simulink model "GridFormingConverter"  (R2024b)
settings: Solver=ode1be  StartTime=0.0  StopTime=simulationTime  FixedStep=gridInverter.vsm.samplingTime  MaxStep=gridInverter.vsm.samplingTime  RelTol=1e-3  AbsTol=1e-3
PreLoadFcn:
  | % Parameterize the model
  | GridFormingConverterInputParameters;
PostLoadFcn:
  | GridFormingConverterTestCondition;
undefined symbols (not defined in the file): base, DiscIntNeverNeededParam, grid, gridInverter, localSolverSampleTime, scrFactorRg, scrFactorXg, transformer, TransmissionLine
libraries: ee_lib x15, eeGeneralControl x15, nesl_utility x11, simulink x5, fl_lib x4, eeTransforms x4, batteryecm_lib x1, eeSinGeneratorThreePhase x1, simulink_extras x1, eePowerMeasurement x1
(part 1 of 3)
CloseFcn:
  | try, close( 'GridFormingConverterNormalOperation'), end
  | try, close( 'GridFormingConverterActivePowerChange'), end
  | try, close( 'GridFormingConverterReactivePowerChange'), end
  | try, close( 'GridFormingConverterGridVoltageChange'), end
  | try, close( 'GridFormingConverterLocalLoadChange'), end
  | try, close( 'GridFormingConverterSmallGridFreqChange'), end
  | try, close( 'GridFormingConverterLargeGridFreqChange'), end
  | try, close( 'GridFormingConverterFullGridFreqChange'), end
  | try, close( 'GridFormingConverter10DegGridPhaseChange'), end
  | try, close( 'GridFormingConverter60DegGridPhaseChange'), end
  | try, close( 'GridFormingConverterPermanentFault'), end
  | try, close( 'GridFormingConverterTemporaryFault'), end
  | try, close( 'GridFormingConverterActivePowerChangeWithRipple'), end
  | try, close( 'GridFormingConverterIslanding'), end
  | try, close( 'GridFormingConverterDampingEffect'), end
  | try, close( 'GridFormingConverterIntertiaEffect'), end
  | try, close('GridFormingConverterVdControllerBodePlot'), end
  | try, close('GridFormingConverterControllerBodePlot'), end
  | try, close( 'GridFormingConverterThreePhaseFault'), end
  | try, close( 'GridFormingConverterThreePhaseFaultStandard'), end
  | try, close( 'GridFormingConverterCompareFaultRideMethod'), end
  | clear base currentLimitMethodSelected expectedSCR
  | clear grid gridInverter primaryBaseImpedance
  | clear realPowerMethodSelected scrSelected scrFactor
  | clear seconadryBaseImpedance shortCircuit
  | clear simulationTime systemSCR testConditionSelected
  | clear testCondition tout transformer TransmissionLine
  | clear gridVoltageProfileVal gridVoltageProfileTime
  | clear gridFrequencyProfileVal gridFrequencyProfileTime
  | clear gridVoltageProfileVal gridVoltageProfileTime
  | clear gridFrequencyProfileVal gridFrequencyProfileTime
  | clear gridPhaseProfileVal gridPhaseProfileTime
  | clear gfmRealPowerRefProfileVal gfmRealPowerRefProfileTime
  | clear gfmControllerRippleInjectMagVal gfmControllerRippleInjectMagTime
  | clear gfmControllerRippleInjectFreqVal gfmControllerRippleInjectFreqTime
  | clear gfmReactivePowerRefProfileVal gfmReactivePowerRefProfileTime
  | clear localLoadRealProfileVal localLoadRealProfileTime
  | clear localLoadReactiveProfileVal localLoadReactiveProfileTime
  | clear faultTriggerVal faultTriggerTime
  | clear circuitBreakerTripSignalVal circuitBreakerTripSignalTime
  | clear disturbanceTime realPartImpedance  localSolverSampleTime
  | clear SimlogGridFormingConverter temprySampleData
  | clear outValue outputTable plotFlag margintable testOutcome
  | clear realPart  XbyRtempFactor scrFactorXg scrFactorRg scrOut XbyROut systemSCR
  | clear outTable marginTable controllerName dampingArray inertiaConstantArray
  | clear imaginaryPart LogsoutGridFormingConverter faultImpedanceArray
  | clear outData
Description:
  | Design and Analysis of Grid-Forming Converter
settings Model: ExtModeTrigDuration=100  Creator=The MathWorks, Inc.  LastModifiedBy=dwx
settings SolverCC: AutoScaleAbsTol=off  AlgebraicLoopSolver=TrustRegion
settings DataIOCC: SaveOutput=off  DSMLogging=off  StateSaveName=tmp_raccel_xout  SignalLoggingName=LogsoutGridFormingConverter  OutputTimes=[0:1.1*3*Voc/(1*2000):1.1*3*Voc/1]  ReturnWorkspaceOutputsName=outData
settings OptimizationCC: ReuseModelBlockBuffer=off  EfficientMapNaN2IntZero=off
settings DebuggingCC: AlgebraicLoopMsg=none  StateNameClashWarn=warning  ArithmeticOperatorsInVariantConditions=warning
settings HardwareCC: ProdBitPerPointer=32  ProdBitPerSizeT=32  ProdBitPerPtrDiffT=32  ProdWordSize=32  ProdHWDeviceType=Intel->x86-32 (Windows32)  TargetBitPerPointer=64  TargetBitPerSizeT=64  TargetBitPerPtrDiffT=64  TargetLongLongMode=on  TargetIntDivRoundTo=Zero  TargetEndianess=LittleEndian  TargetWordSize=64  TargetHWDeviceType=MATLAB Host  ProdEqTarget=off
settings ModelReferenceCC: EnableRefExpFcnMdlSchedulingChecks=on  PropagateSignalLabelsOutOfModel=off
settings SFSimCC: CustomCodeUndefinedFunction=UseInterfaceOnly
settings RTWCC: SystemTargetFile=raccel.tlc  TemplateMakefile=raccel_default_tmf  RTWVerbose=off  RTWUseSimCustomCode=on  GPUComputeCapability=3.5
settings CodeAppCC: GenerateComments=off  MaxIdLength=128  SimulinkBlockComments=off
settings RaccelTargetCC: TargetLangStandard=C99 (ISO)  InstructionSetFMA=off  OptimizeReductions=off  LogToMDFFile=off  ENABLE_SLEXEC_SSBRIDGE=1  RTWCAPIParams=on  RTWCAPIRootIO=on
settings SimscapeCC: SimscapeLogType=all  SimscapeLogSimulationStatistics=on  SimscapeLogName=SimlogGridFormingConverter  SimscapeLogLimitData=off

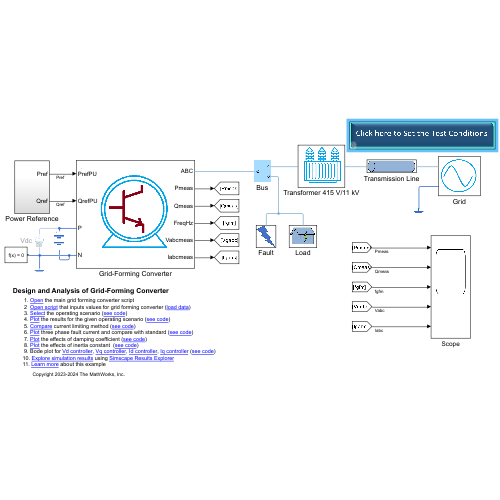
[thumbnail: Simulink's stored preview of the top-level diagram]
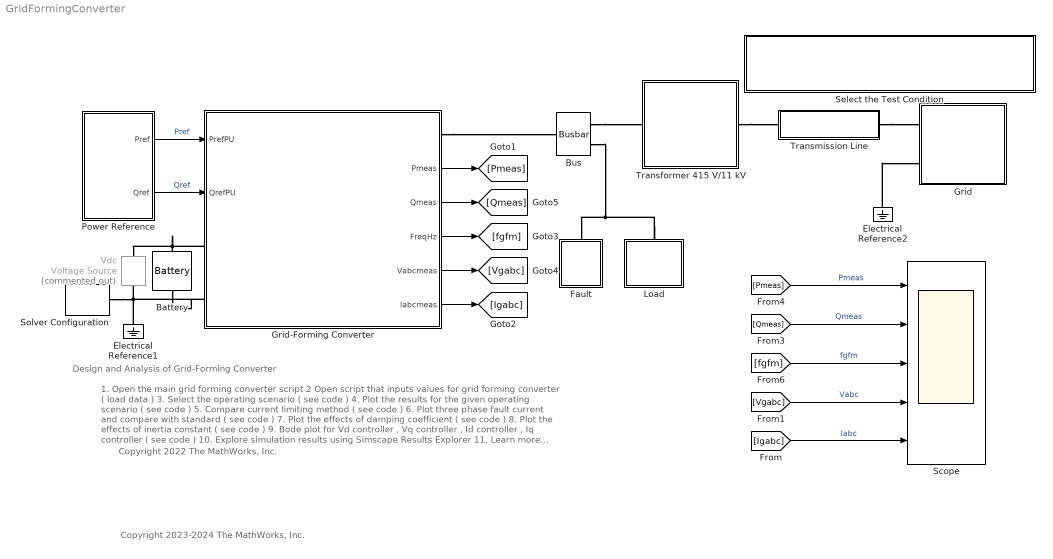
== system GridFormingConverter ==
  note: Copyright 2023-2024 The MathWorks, Inc.
  note: 1. Open the main grid forming converter script
      | 2 Open script that inputs values for grid forming converter ( load data )
      | 3. Select the operating scenario ( see code )
      | 4. Plot the results for the given operating scenario ( see code )
      | 5. Compare current limiting method ( see code )
      | 6. Plot three phase fault current and compare with standard ( see code )
      | 7. Plot the effects of damping coefficient ( see code )
      | 8. Plot the effects of inertia constant ( see code )
      | 9. Bode plot for Vd controller , Vq controller , Id controller , Iq controller ( see code )
      | 10. Explore simulation results using Simscape Results Explorer
      | 11. Learn more about this example
  note: Design and Analysis of Grid-Forming Converter
  note: Copyright 2022 The MathWorks, Inc.
  Battery : batteryecm_lib/Battery  Vnom=battery.vbat_nominal V  prm_dir=simscape.enum.battery.prm_dir.disabled  R1_dis=2 Ohm  R1_ch=2 Ohm  R1=battery.resistance Ohm  prm_AH=simscape.enum.battery.prm_AH.finite  AH=battery.capacity A*hr  V1=battery.vbat_1 V  AH1=battery.charge_vbat1 A*hr  prm_R2=simscape.enum.battery.prm_R2.disabled  R2=2000 Ohm  Tmeas=298.15 K  charge_measurement_port=simscape.enum.battery.enable.no  prm_dyn=simscape.enum.battery.prm_dyn.off  Rp1=0.005 Ohm  tau1=30 s  Rp2=0.005 Ohm  tau2=30 s  Rp3=0.005 Ohm  tau3=30 s  Rp4=0.005 Ohm  tau4=30 s  Rp5=0.005 Ohm  tau5=30 s  prm_fade=simscape.enum.battery.prm_fade.disabled  N_fade=100  AH_fade=45 A*hr  R1_fade=2.02 Ohm  R1_ch_fade=2.02 Ohm  V1_fade=10.35 V  prm_age=simscape.enum.battery.prm_age.disabled  prm_age_OCV=simscape.enum.battery.prm_age_OCV.OCV  OCV_age=0.9  SOC_age=60  Tmeas_age=298.15 K  delta_time_age_vec=[0] d  temperature_age_vec=[273] K  OCV_scaling_age=2.2134e6  OCV_offset_age=1.632e6  temp_exp_age=0.515833569 V  t_exp_age=0.75  Vnom_T2=12 V  R1_T2=2.2 Ohm  R1_T2_dis=2.2 Ohm  R1_T2_ch=2.2 Ohm  V1_T2=11.4 V  R2_T2=2200 Ohm  Rp1_T2=0.005 Ohm  tau1_T2=30 s  Rp2_T2=0.005 Ohm  tau2_T2=30 s  Rp3_T2=0.005 Ohm  tau3_T2=30 s  Rp4_T2=0.005 Ohm  tau4_T2=30 s  Rp5_T2=0.005 Ohm  tau5_T2=30 s  Tmeas2=273.15 K  thermal_port=simscape.enum.thermaleffects.omit  thermal_mass=30000 J/K  i_specify=off  i_priority=None  i=0 A  i_nominal_specify=off  i_nominal_value=1  i_nominal_unit=A  v_specify=off  v_priority=None  v=0 V  v_nominal_specify=off  v_nominal_value=1  v_nominal_unit=V  charge_specify=off  charge_priority=High  charge=50 A*hr  charge_nominal_specify=off  charge_nominal_value=1  charge_nominal_unit=A*hr  num_cycles_specify=off  num_cycles_priority=High  num_cycles=0  num_cycles_nominal_specify=off  num_cycles_nominal_value=1  num_cycles_nominal_unit=1  temperature_specify=off  temperature_priority=High  temperature=298.15 K  temperature_nominal_specify=off  temperature_nominal_value=1  temperature_nominal_unit=K
  Bus : ee_lib/Connectors & References/Busbar  n_nodes=ee.enum.connectors.busbar_number_of_connections.three  VRated=gridInverter.lineRMSVoltage V  freq=gridInverter.frequency Hz  show_ps=ee.enum.connectors.busbar_measurement.false
      settings: AttributesFormatString=%<Tag>  InternalSimscapePortConfiguration="{\"Bottom\":[],\"Left\":[{\"id\":\"N1\",\"label\":\"~1\",\"type\":\"foundation.electrical.three_phase\"},{\"id\":\"N3\",\"label\":\"~3\",\"type\":\"foundation.electrical.three_phase\"}],\"Right\":[{\"id\":\"N2\",\"label\":\"~2\",\"type\":\"foundation.electrical.three_phase\"}],\"Top\":[]}"
  Electrical Reference1 : fl_lib/Electrical/Electrical Elements/Electrical Reference
  Electrical Reference2 : fl_lib/Electrical/Electrical Elements/Electrical Reference
  Fault : Subsystem
      mask Display: image('$imagefile'); % Use "Edit Image" on toolstrip to change.
  Grid : Subsystem
      mask Display: image('$imagefile'); % Use "Edit Image" on toolstrip to change.
  Grid-Forming Converter : Subsystem
      settings: PortSchema="{\"entries\":[{\"content\":{\"sides\":[{\"content\":{\"connectorIds\":[\"In1\",\"In2\",\"LConn1\",\"LConn2\"]},\"type\":\"ConnectorPlacement.EquallySpacedRectSide\",\"uuid\":\"d0fa63af-a5a8-4d4b-b4c3-664fd5bcaa8a\"},{\"content\":{\"connectorIds\":[\"RConn1\",\"Out1\",\"Out2\",\"Out3\",\"Out4\",\"Out5\"],\"side\":\"RIGHT\"},\"type\":\"ConnectorPlacement.EquallySpacedRectSide\",\"uuid\":\"972b6ea6-c710-49ff-8fe7-d9d32c573dae\"},{\"content\":{\"connectorIds\":[],\"side\":\"TOP\"},\"type\":\"ConnectorPlacement.EquallySpacedRectSide\",\"uuid\":\"eb20b8c4-85b6-4776-9f5e-c8dafbcbb9bc\"}]},\"type\":\"ConnectorPlacement.EquallySpacedConnector\",\"uuid\":\"e08a9662-8437-4e94-9fe5-abd27988c7a0\"}],\"packageUris\":[\"http://schema.mathworks.com/mf0/Connector/R2020b\"],\"version\":\"1.0\"}"
      mask Display: image('$imagefile'); % Use "Edit Image" on toolstrip to change.
  Load : Subsystem
      mask Display: image('$imagefile'); % Use "Edit Image" on toolstrip to change.
  Power Reference : Subsystem
  Scope : Scope  NumInputPorts=5
  Select the Test Condition : Subsystem  mask(Set the Test Conditions){scrParameter=2.5, XbyRRatio=4, testCondition=Change in grid frequency 2Hz/s, +2Hz and 1Hz/s till -5Hz, realPowerControl=Virtual Synchronous Machine, currentLimitControl=Current Limiting}
      mask prompts: scrParameter "Grid short circuit ratio"; XbyRRatio "Grid X/R ratio"; testCondition "Test condition"; realPowerControl "Active power control"; currentLimitControl "Current limiting control"
      mask help: This blocks helps to setup the test condition variables, test scenario, simulate the model and plot the results.
      mask Help: This blocks helps to setup the test condition variables, test scenario, simulate the model and plot the results.
      mask TypeOptions testCondition: Normal operation | Change in active power reference | Change in reactive power reference | Change in grid voltage | Change in local load | Change in grid frequency 1Hz/s, +0.5Hz | Change in grid frequency 2Hz/s, +2Hz | Change in grid frequency 2Hz/s, +2Hz and 1Hz/s till -5Hz | Change in grid phase by 10 degrees | Change in grid phase by 60 degrees | Permanent three-phase fault | Temporary three-phase fault | Islanding condition
      mask TypeOptions realPowerControl: Virtual Synchronous Machine | Droop control
      mask TypeOptions currentLimitControl: Virtual Impedance | Current Limiting | Virtual Impedance and Current Limiting
      mask DialogControl testCon Prompt: Provide test condition parameters
      mask DialogControl testCon Callback: edit GridFormingConverterTestCondition
      mask DialogControl applyParameters Prompt: Apply the test condition parameters into the model
      mask DialogControl applyParameters Callback:
      | run('GridFormingConverterInputParameters.mlx');
      | 
      | 
      |     % Setting the proper short circuit ratio
      |     testCondition.SCR = str2double(get_param(gcb,'scrParameter'));
      |     testCondition.XbyR = str2double(get_param(gcb,'XbyRRatio'));
      | 
      |     % Setting the Test condition
      |     testCondition.testCondition = get_param(gcb,'testCondition');
      |    % testCondition.scrSelected =  get_param(gcb,'scrRange');
      |     testCondition.currentLimitMethod = get_param(gcb,'currentLimitControl');
      |     testCondition.activePowerMethod = get_param(gcb,'realPowerControl');
      | 
      |     run('GridFormingConverterTestCondition.mlx');
      |     assignin('base','simulationTime',simulationTime);
      |     assignin('base','localSolverSampleTime',localSolverSampleTime);
      |     assignin('base','scrFactorRg',scrFactorRg);
      |     assignin('base','scrFactorXg',scrFactorXg);
      | 
      |     set_param([bdroot,'/Grid-Forming Converter/Grid-Forming Converter Control'],'powerControl',testCondition.activePowerMethod);
      |     set_param([bdroot,'/Grid-Forming Converter/Grid-Forming Converter Control'],'currentLimit',testCondition.currentLimitMethod);
      | 
      |     assignin('base','testCondition',testCondition);
      mask DialogControl simulate Prompt: Simulate the test condition
      mask DialogControl simulate Callback:
      | % Auto applying the mask dialog
      |     dlg = DAStudio.ToolRoot.getOpenDialogs();
      |     dlg = dlg.find('dialogTag','SubSystem.Set_the_Test_Conditions');
      |     imd = DAStudio.imDialog.getIMWidgets(dlg);
      |     imd.clickOk(dlg);
      | 
      |     % Inputting the grid-forming converter parameters
      |     run('GridFormingConverterInputParameters.mlx');
      | 
      | 
      |     % Setting the proper short circuit ratio
      |     testCondition.SCR = str2double(get_param(gcb,'scrParameter'));
      |     testCondition.XbyR = str2double(get_param(gcb,'XbyRRatio'));
      | 
      | 
      |     % Setting the Test condition
      |     testCondition.testCondition = get_param(gcb,'testCondition');
      |     %testCondition.scrSelected =  get_param(gcb,'scrRange');
      | 
      |     run('GridFormingConverterTestCondition.mlx');
      |     assignin('base','simulationTime',simulationTime);
      |     assignin('base','localSolverSampleTime',localSolverSampleTime);
      |     assignin('base','scrFactorRg',scrFactorRg);
      |     assignin('base','scrFactorXg',scrFactorXg);
      | 
      |     % Setting current limit and real power method
      |     testCondition.currentLimitMethod = get_param(gcb,'currentLimitControl');
      |     testCondition.activePowerMethod = get_param(gcb,'realPowerControl');
      |     set_param([bdroot,'/Grid-Forming Converter/Grid-Forming Converter Control'],'powerControl',testCondition.activePowerMethod);
      |     set_param([bdroot,'/Grid-Forming Converter/Grid-Forming Converter Control'],'currentLimit',testCondition.currentLimitMethod);
      | 
      |     assignin('base','testCondition',testCondition);
      | 
      |     % Simulating the model
      |     open_system([bdroot,'/Scope']);
      |     %sim(bdroot,'SrcWorkspace','base');
      |     outputTable = PlotGridFormingConverter(testCondition,1);
      mask Display: image('$imagefile'); % Use "Edit Image" on toolstrip to change.
  Solver Configuration : nesl_utility/Solver Configuration  PhysicalDomain=network_engine_domain  SubClassName=solver  LeftPortType=input  RightPortType=generic  Tones=[]  Harmonics=[]  SimulateNoise=off  Profile=off  UseLocalSampling=off  EnableSwitchedLinearOptims=on  FrequencyDomain=off  UseCCode=off  RelTol=0.001  AbsTol=1e-06  MinStep=1e-09  ToWorkspace=off  RevertToSquareIcSolve=off  NumHomotopyIterations=100  PhasorMode=off  PhasorModeNumHarmonics=1  ConsistencySolver=NEWTON_FTOL  IndexReductionMethod=DerivativeReplacement  DoDC=off  ResidualTolerance=1e-09  ConsistencyTolSource=GLOBAL  ConsistencyAbsTol=0.001  ConsistencyRelTol=0.001  ConsistencyTolFactor=0.001  UseLocalSolver=on  LocalSolverChoice=NE_BACKWARD_EULER_ADVANCER  ResolveIndetEquations=on  FunctionEvalNumThread=1  LocalSolverSampleTime=localSolverSampleTime  DoFixedCost=on  MaxNonlinIter=3  MaxModeIter=2  ComputeImpulses=off  ImpulseIterations=2  LinearAlgebra=auto  LinearAlgebraNumThread=0  EquationFormulation=NE_TIME_EF  DelaysMemoryBudget=1024  AutomaticFiltering=on  FilteringTimeConstant=0.001  PartitionStorageMethod=AS_NEEDED  PartitionMemoryBudget=1024  PartitionMethod=ROBUST  MultibodyUseLocalSolver=off  MultibodyLocalSolverChoice=ODE1  MultibodyLocalSolverSampleTime=0.001
  Transformer 415 V/11 kV : Subsystem
      mask Display: image('$imagefile'); % Use "Edit Image" on toolstrip to change.
  Transmission Line : Subsystem
      mask Display: image('$imagefile'); % Use "Edit Image" on toolstrip to change.
  Vdc : ee_lib/Sources/Voltage Source  Commented=on  dc_voltage=gridInverter.DCVoltage V  ac_voltage=0 V  ac_shift=0 rad  ac_frequency=0 Hz  noise_mode=ee.enum.sources.noise.Disabled  PSD=0 V^2/Hz  sample_time=1e-3 s  repeatability=ee.enum.sources.repeatability.NotRepeatable  user_seed=0  auto_seed=3499211588  i_specify=off  i_priority=None  i=0 A  i_nominal_specify=off  i_nominal_value=1  i_nominal_unit=A  v_specify=off  v_priority=None  v=0 V  v_nominal_specify=off  v_nominal_value=1  v_nominal_unit=V
  wires:
  [Pmeas] -> Scope/1  "Pmeas"
  [Qmeas] -> Scope/2  "Qmeas"
  [fgfm] -> Scope/3  "fgfm"
  [Vgabc] -> Scope/4  "Vabc"
  [Igabc] -> Scope/5  "Iabc"
  Power Reference/1(Pref) -> Grid-Forming Converter/1(PrefPU)  "Pref"
  Power Reference/2(Qref) -> Grid-Forming Converter/2(QrefPU)  "Qref"
  Grid-Forming Converter/1(Pmeas) -> [Pmeas]
  Grid-Forming Converter/2(Qmeas) -> [Qmeas]
  Grid-Forming Converter/3(FreqHz) -> [fgfm]
  Grid-Forming Converter/5(Iabcmeas) -> [Igabc]
  Grid-Forming Converter/4(Vabcmeas) -> [Vgabc]
  connections:
  Electrical Reference2/LConn1 -- Grid/LConn2
  Bus/LConn1 -- Transformer 415 V/11 kV/LConn1
  Bus/LConn2 -- Load/LConn1 -- Fault/LConn1
  Transformer 415 V/11 kV/RConn1 -- Transmission Line/LConn1
  Transmission Line/RConn1 -- Grid/LConn1
  Grid-Forming Converter/LConn1 -- Battery/LConn1 -- Vdc/LConn1
  Electrical Reference1/LConn1 -- Battery/RConn1 -- Grid-Forming Converter/LConn2 -- Solver Configuration/RConn1 -- Vdc/RConn1
  Grid-Forming Converter/RConn1 -- Bus/RConn1

== system GridFormingConverter/Fault ==
  Fault : ee_lib/Utilities/Fault (Three-Phase)  fault_type_option=11  R_pn_fault=testCondition.faultResistance Ohm  R_ng_fault=1e-3 Ohm  exposemeasurement=ee.enum.exposemeasurement.hidden  enable_external_fault=ee.enum.external_fault.visible  fault_threshold=0.5  fault_condition=1  fault_resettable=1  enable_temporal_fault=0  fault_start_time=1 s  fault_duration=0.1 s  G_parasitic=1e-5 1/Ohm
      settings: InternalSimscapePortConfiguration="{\"Bottom\":[],\"Left\":[{\"id\":\"N\",\"label\":\"~\",\"type\":\"foundation.electrical.three_phase\"},{\"id\":\"F\",\"label\":\"F\",\"type\":\"input\"}],\"Right\":[],\"Top\":[]}"
  Fault trigger : FromWorkspace  VariableName=testCondition.faultTrigger  SampleTime=localSolverSampleTime  Interpolate=off  ZeroCross=off  OutputAfterFinalValue=Holding final value
  Simulink-PS Converter1 : nesl_utility/Simulink-PS Converter  PhysicalDomain=network_engine_domain  SubClassName=ps_input  LeftPortType=input  RightPortType=output  PseudoPeriodic=off  Frequencies=[]  NoiseDistribution=none  NoiseParameters=[]  Unit=1  AffineConversion=off  FilteringAndDerivatives=provide  SimscapeFilterOrder=1  InputFilterTimeConstant=0.001  UdotUserProvided=0
  abc : PMIOPort  Side=Left
  wires:
  Fault trigger/1 -> Simulink-PS Converter1/1  "faultSignal"
  connections:
  Fault/LConn2 -- Simulink-PS Converter1/RConn1
  Fault/LConn1 -- abc/RConn1

== system GridFormingConverter/Grid ==
  Gain : Gain  Gain=1.05*grid.gridVoltageLL*sqrt(2/3)
  Grid : ee_lib/Sources/Controlled Voltage Source (Three-Phase)  input_option=ee.enum.inputType.instantaneous  FRated=60 Hz
      settings: InternalSimscapePortConfiguration="{\"Bottom\":[],\"Left\":[{\"id\":\"S\",\"label\":\"S\",\"type\":\"input\"},{\"id\":\"n\",\"label\":\"n\",\"type\":\"foundation.electrical.electrical\"}],\"Right\":[{\"id\":\"N\",\"label\":\"~\",\"type\":\"foundation.electrical.three_phase\"}],\"Top\":[]}"
  Grid frequency : FromWorkspace  VariableName=testCondition.gridFrequencyProfile  SampleTime=localSolverSampleTime  OutputAfterFinalValue=Holding final value
  Grid voltage magnitude : FromWorkspace  VariableName=testCondition.gridVoltageProfile  SampleTime=localSolverSampleTime  Interpolate=off  OutputAfterFinalValue=Holding final value
  Grid voltage phase : FromWorkspace  VariableName=testCondition.gridPhaseProfile  SampleTime=localSolverSampleTime  Interpolate=off  OutputAfterFinalValue=Holding final value
  Simulink-PS Converter1 : nesl_utility/Simulink-PS Converter  PhysicalDomain=network_engine_domain  SubClassName=ps_input  LeftPortType=input  RightPortType=output  PseudoPeriodic=off  Frequencies=[]  NoiseDistribution=none  NoiseParameters=[]  Unit=1  AffineConversion=off  FilteringAndDerivatives=provide  SimscapeFilterOrder=1  InputFilterTimeConstant=0.001  UdotUserProvided=0
  Sine Wave Generator (Three-Phase) : eeSinGeneratorThreePhase/Sine Wave Generator (Three-Phase)  Ts=localSolverSampleTime
  Source impedance : ee_lib/Passive/RLC Assemblies/RLC (Three-Phase)  port_option=ee.enum.threePhasePort.composite  component_structure=ee.enum.rlc.structure.SeriesRL  R=grid.gridResistance*scrFactorRg Ohm  L=grid.gridInductance*scrFactorXg H  C=1e-6 F  R_parasitic=0 Ohm  G_parasitic=0 1/Ohm  IL_specify=off  IL_priority=High  IL=[0, 0, 0] A  IL_nominal_specify=off  IL_nominal_value=1  IL_nominal_unit=A  VC_specify=off  VC_priority=High  VC=[0, 0, 0] V  VC_nominal_specify=off  VC_nominal_value=1  VC_nominal_unit=V
      settings: InternalSimscapePortConfiguration="{\"Bottom\":[],\"Left\":[{\"id\":\"N1\",\"label\":\"~1\",\"type\":\"foundation.electrical.three_phase\"}],\"Right\":[{\"id\":\"N2\",\"label\":\"~2\",\"type\":\"foundation.electrical.three_phase\"}],\"Top\":[]}"
  Terminator : Terminator
  P : PMIOPort  Side=Left
  N : PMIOPort  Port=2  Side=Left
  wires:
  Sine Wave Generator (Three-Phase)/1 -> Simulink-PS Converter1/1
  Grid voltage phase/1 -> Sine Wave Generator (Three-Phase)/2  "GridPhase"
  Sine Wave Generator (Three-Phase)/2 -> Terminator/1
  Grid voltage magnitude/1 -> Gain/1  "GridMag"
  Gain/1 -> Sine Wave Generator (Three-Phase)/1
  Grid frequency/1 -> Sine Wave Generator (Three-Phase)/3  "GridFreq"
  connections:
  Grid/LConn1 -- Simulink-PS Converter1/RConn1
  Grid/LConn2 -- N/RConn1
  Source impedance/LConn1 -- Grid/RConn1
  Source impedance/RConn1 -- P/RConn1

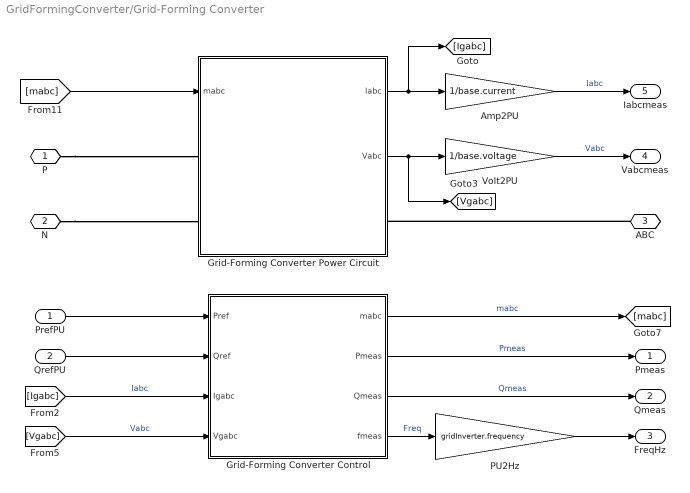
== system GridFormingConverter/Grid-Forming Converter ==
  PrefPU : Inport
  QrefPU : Inport  Port=2
  Amp2PU : Gain  Gain=1/base.current
  Grid-Forming Converter Control : Subsystem  mask(Grid-Forming Controller){power=gridInverter.apparentPower*1e3, gridLineVoltage=gridInverter.lineRMSVoltage, powerFreq=gridInverter.frequency, dcBusVoltage=gridInverter.DCVoltage, measSampleTime=gridInverter.measurementSampleTime, powerControl=Virtual Synchronous Machine, activePowerSampleTime=gridInverter.droopControl.sampleTime, droopSlope=gridInverter.droopControl.freqSlopeMp, droopT1=gridInverter.droopControl.T1, droopT2=gridInverter.droopControl.T2, droopTC=gridInverter.droopControl.lpfTimeConst, vsmPmeasFilterTC=gridInverter.vsm.PmeasTimeConst, vsmFreqDroop=gridInverter.vsm.freqDroop, vsmInertiaTC=gridInverter.vsm.inertiaConstant, vsmDampingConst=gridInverter.vsm.dampingCoefficent, dampingPowerMaxLimit=gridInverter.vsm.maxDampingPower, dampingPowerMinLimit=gridInverter.vsm.minDampingPower, freqMeasTimeConst=gridInverter.freqMeasTimeConst, freqOption=Grid Frequency Measurement, voltreference=gridInverter.Qcontrol.voltageReference, QVoltFilterTC=gridInverter.Qcontrol.QmeasTimeConst, QVoltDroop=gridInverter.Qcontrol.voltageDroop, lowVoltageSupportGain=gridInverter.Qcontrol.lowVoltageSupportGain, currentLimit=Current Limiting, maxSatCurrentLimit=gridInverter.currentLimit.maxSaturationCurrent, maxVICurrentLimit=gridInverter.currentLimit.viCurrentLimit, ctLimitVirtualImp=gridInverter.currentLimit.virImpResistanceCoeff, ctLimitXbyR=gridInverter.currentLimit.virImpXbyR, ctLimitDelayTime=gridInverter.currentLimit.maxSaturationDelay, currentSatTime=gridInverter.currentLimit.satCurrentRunTime, currentVITimeConst=gridInverter.currentLimit.viFilterTimeConst, modeTransferTime=10*gridInverter.controller.CurrentControlSampleTime, voltControlTs=gridInverter.controller.VoltageControlSampleTime, vdPGain=gridInverter.controller.voltControllerKp, VdIGain=gridInverter.controller.voltControllerKi, VdMaxCt=gridInverter.controller.voltageMaxId, VdMinCt=gridInverter.controller.voltageMinId, VqPGain=gridInverter.controller.voltControllerKp, VqIGain=gridInverter.controller.voltControllerKi, VqMaxCt=gridInverter.controller.voltageMaxIq, VqMinCt=gridInverter.controller.voltageMinIq, vdvqLPFTimeConst=gridInverter.controller.voltMeasTimeConst, currentControlTs=gridInverter.controller.CurrentControlSampleTime, filterInductance=gridInverter.L, IdPGain=gridInverter.controller.ctControllerKp, IdIGain=gridInverter.controller.ctControllerKi, IqPGain=gridInverter.controller.ctControllerKp, IqIGain=gridInverter.controller.ctControllerKi}
      mask prompts: power "Grid-forming converter power (VA)"; gridLineVoltage "Grid line voltage (V)"; powerFreq "Grid frequency (Hz)"; dcBusVoltage "DC bus voltage (V)"; measSampleTime "Measurement sample time (s)"; powerControl "Active Power Control"; activePowerSampleTime "Power controller sample time (s)"; droopSlope "Power droop slope (pu, Hz/W)"; droopT1 "Lead-Lag numerator time constant (s)"; droopT2 "Lead-Lag denominator time constant (s)"; droopTC "Filter cut-off time constant (s)"; vsmPmeasFilterTC "Power measurement filter time constant (s)"; vsmFreqDroop "Frequency droop (pu,  W/Hz)"; vsmInertiaTC "Inertia constant M (pu)"; vsmDampingConst "Damping constant (pu/Hz)"; dampingPowerMaxLimit "Damping power maximum limit (pu)"; dampingPowerMinLimit "Damping power minimum limit (pu)"; freqMeasTimeConst "Frequency measurement time constant (s)"; freqOption "Damping power frequency option"; voltreference "Voltage reference value (pu)"; QVoltFilterTC "Power measurement filter time constant (s)"; QVoltDroop "Voltage droop (pu, V/VAr)"; lowVoltageSupportGain "Low voltage support gain (pu, A/V)"; currentLimit "Current limiting method"; maxSatCurrentLimit "Maximum current saturation (pu)"; maxVICurrentLimit "Maximum virtual impedance current (pu)"; ctLimitVirtualImp "Virtual impedance coefficient (pu.Ohm/pu.A)"; ctLimitXbyR "Virtual X/R ratio"; ctLimitDelayTime "Maximum current delay time (s)"; currentSatTime "Current limiting run time (s)"; currentVITimeConst "Filter time constant (s)"; modeTransferTime "Mode transfer time (s)"; voltControlTs "Voltage controller sample time (s)"; vdPGain "Vd proportional gain"; VdIGain "Vd integral gain"; VdMaxCt "Vd maximum current limit (A)"; VdMinCt "Vd minimum current limit (A)"; VqPGain "Vq proportional gain"; VqIGain "Vq integral gain"; VqMaxCt "Vq maximum current limit (A)"; VqMinCt "Vq minimum current limit (A)"; vdvqLPFTimeConst "Voltage measurement filter time constant (s)"; currentControlTs "Current controller sample time (s)"; filterInductance "Filter inductance (H)"; IdPGain "Id proportional gain"; IdIGain "Id integral gain"; IqPGain "Iq proportional gain"; IqIGain "Iq integral gain"
      mask help: This block implements the grid forming controller with fault ride through capability. Input to the controller are active and reactive power reference in per unit and the sensed three-phase phase current in amphere and phase voltage in volts.
      mask init:
      | powerChoice = get_param(gcb,'powerControl');
      | currentChoice = get_param(gcb,'currentLimit');
      | 
      | powerloc = [gcb, '/Power Control/ActivePowerControl']; 
      | currentloc = [gcb, '/Current Limiting/CurrentLimitingMethod'];
      | freqLoc = [gcb,'/Power Control/ActivePowerControl/vsmControl/Damping Frequency'];
      | 
      | switch powerChoice
      |     case 'Virtual Synchronous Machine'
      |         set_param(powerloc, 'LabelModeActiveChoice', 'vsm');
      |         dampingFreqChoice = get_param(gcb,'freqOption');
      |         if strcmp(dampingFreqChoice,'Grid Frequency Measurement')
      |             set_param(freqLoc, 'LabelModeActiveChoice', 'freqMeas');
      |         else
      |             set_param(freqLoc, 'LabelModeActiveChoice', 'constFreq');
      |         end
      |     case 'Droop Control'
      |          set_param(powerloc, 'LabelModeActiveChoice', 'droop');
      |    otherwise
      |         disp('Choose proper active power control method')
      | end
      | switch currentChoice
      |     case 'Virtual Impedance'
      |           set_param(currentloc, 'LabelModeActiveChoice', 'virimp');
      |     case 'Current Limiting'
      |          set_param(currentloc, 'LabelModeActiveChoice', 'ctSat');
      |     case 'Virtual Impedance and Current Limiting'
      |             set_param(currentloc, 'LabelModeActiveChoice', 'both');
      |     otherwise
      |         disp('Choose proper current limiting method')
      | end
      mask Help: This block implements the grid forming controller with fault ride through capability. Input to the controller are active and reactive power reference in per unit and the sensed three-phase phase current in amphere and phase voltage in volts.
      mask TypeOptions powerControl: Virtual Synchronous Machine | Droop Control
      mask Callback powerControl:
      | h = Simulink.Mask.get(gcb);
      | slectedActivePowerControl=get_param(gcb,'powerControl');
      | %slectedActivePowerControl = h.Parameters(find(string({h.Parameters.Name}) == 'powerControl')).Value;
      | switch slectedActivePowerControl
      |     case 'Virtual Synchronous Machine'
      |         h.Parameters(find(string({h.Parameters.Name}) == 'droopSlope')).Visible = 'off';
      |         h.Parameters(find(string({h.Parameters.Name}) == 'droopTC')).Visible = 'off';
      |         h.Parameters(find(string({h.Parameters.Name}) == 'droopT1')).Visible = 'off';
      |         h.Parameters(find(string({h.Parameters.Name}) == 'droopT2')).Visible = 'off';
      |         h.Parameters(find(string({h.Parameters.Name}) == 'vsmPmeasFilterTC')).Visible = 'on';
      |         h.Parameters(find(string({h.Parameters.Name}) == 'vsmFreqDroop')).Visible = 'on';
      |         h.Parameters(find(string({h.Parameters.Name}) == 'vsmInertiaTC')).Visible = 'on';
      |         h.Parameters(find(string({h.Parameters.Name}) == 'vsmDampingConst')).Visible = 'on';
      |         h.Parameters(find(string({h.Parameters.Name}) == 'dampingPowerMaxLimit')).Visible = 'on';
      |         h.Parameters(find(string({h.Parameters.Name}) == 'dampingPowerMinLimit')).Visible = 'on';
      |         h.Parameters(find(string({h.Parameters.Name}) == 'freqOption')).Visible = 'on';
      |         h.Parameters(find(string({h.Parameters.Name}) == 'freqMeasTimeConst')).Visible = 'on';
      |     case 'Droop Control'
      |         h.Parameters(find(string({h.Parameters.Name}) == 'droopSlope')).Visible = 'on';
      |         h.Parameters(find(string({h.Parameters.Name}) == 'droopTC')).Visible = 'on';
      |         h.Parameters(find(string({h.Parameters.Name}) == 'droopT1')).Visible = 'on';
      |         h.Parameters(find(string({h.Parameters.Name}) == 'droopT2')).Visible = 'on';
      |         h.Parameters(find(string({h.Parameters.Name}) == 'vsmPmeasFilterTC')).Visible = 'off';
      |         h.Parameters(find(string({h.Parameters.Name}) == 'vsmFreqDroop')).Visible = 'off';
      |         h.Parameters(find(string({h.Parameters.Name}) == 'vsmInertiaTC')).Visible = 'off';
      |         h.Parameters(find(string({h.Parameters.Name}) == 'vsmDampingConst')).Visible = 'off';
      |         h.Parameters(find(string({h.Parameters.Name}) == 'dampingPowerMaxLimit')).Visible = 'off';
      |         h.Parameters(find(string({h.Parameters.Name}) == 'dampingPowerMinLimit')).Visible = 'off';
      |         h.Parameters(find(string({h.Parameters.Name}) == 'freqOption')).Visible = 'off';
      |         h.Parameters(find(string({h.Parameters.Name}) == 'freqMeasTimeConst')).Visible = 'on';
      | 
      |     otherwise
      |         disp('Choose proper active power control method')
      | end
      mask TypeOptions freqOption: Grid Frequency Measurement | Constant Frequency Reference
      mask TypeOptions currentLimit: Virtual Impedance | Current Limiting | Virtual Impedance and Current Limiting
      mask Callback currentLimit:
      | h = Simulink.Mask.get(gcb);
      | currentLimitControl=get_param(gcb,'currentLimit');
      | %slectedActivePowerControl = h.Parameters(find(string({h.Parameters.Name}) == 'powerControl')).Value;
      | switch currentLimitControl
      |     case 'Virtual Impedance'
      |         h.Parameters(find(string({h.Parameters.Name}) == 'maxVICurrentLimit')).Visible = 'on';
      |         h.Parameters(find(string({h.Parameters.Name}) == 'ctLimitVirtualImp')).Visible = 'on';
      |         h.Parameters(find(string({h.Parameters.Name}) == 'ctLimitXbyR')).Visible = 'on';
      |         h.Parameters(find(string({h.Parameters.Name}) == 'maxSatCurrentLimit')).Visible = 'off';
      |         h.Parameters(find(string({h.Parameters.Name}) == 'ctLimitDelayTime')).Visible = 'off';
      |         h.Parameters(find(string({h.Parameters.Name}) == 'currentSatTime')).Visible = 'off';
      |         h.Parameters(find(string({h.Parameters.Name}) == 'currentVITimeConst')).Visible = 'on';
      |         h.Parameters(find(string({h.Parameters.Name}) == 'modeTransferTime')).Visible = 'off';
      | 
      | 
      |     case 'Current Limiting'
      |         h.Parameters(find(string({h.Parameters.Name}) == 'maxVICurrentLimit')).Visible = 'off';
      |         h.Parameters(find(string({h.Parameters.Name}) == 'ctLimitVirtualImp')).Visible = 'off';
      |         h.Parameters(find(string({h.Parameters.Name}) == 'ctLimitXbyR')).Visible = 'off';
      |         h.Parameters(find(string({h.Parameters.Name}) == 'maxSatCurrentLimit')).Visible = 'on';
      |         h.Parameters(find(string({h.Parameters.Name}) == 'ctLimitDelayTime')).Visible = 'on';
      |         h.Parameters(find(string({h.Parameters.Name}) == 'currentSatTime')).Visible = 'off';
      |         h.Parameters(find(string({h.Parameters.Name}) == 'currentVITimeConst')).Visible = 'off';
      |         h.Parameters(find(string({h.Parameters.Name}) == 'modeTransferTime')).Visible = 'off';
      | 
      |     case 'Virtual Impedance and Current Limiting'
      |         h.Parameters(find(string({h.Parameters.Name}) == 'maxVICurrentLimit')).Visible = 'on';
      |         h.Parameters(find(string({h.Parameters.Name}) == 'ctLimitVirtualImp')).Visible = 'on';
      |         h.Parameters(find(string({h.Parameters.Name}) == 'ctLimitXbyR')).Visible = 'on';
      |         h.Parameters(find(string({h.Parameters.Name}) == 'maxSatCurrentLimit')).Visible = 'on';
      |         h.Parameters(find(string({h.Parameters.Name}) == 'ctLimitDelayTime')).Visible = 'off';
      |         h.Parameters(find(string({h.Parameters.Name}) == 'currentSatTime')).Visible = 'on';
      |         h.Parameters(find(string({h.Parameters.Name}) == 'currentVITimeConst')).Visible = 'on';
      |         h.Parameters(find(string({h.Parameters.Name}) == 'modeTransferTime')).Visible = 'on';
      | 
      |     otherwise
      |         disp('Choose proper current limiting method')
      | end
      mask DialogControl ParameterGroupVar Prompt: Grid-Forming Controller Parameters
      mask DialogControl GFMGroup Prompt: Grid-Forming Converter Specifications
      mask DialogControl Pcontrolgrp Prompt: Active Power Controller Parameters
      mask DialogControl QcontrolGrp Prompt: Reactive Power Controller Parameters
      mask DialogControl faultRideThroughGrp Prompt: Fault Ride-Through Parameters
      mask DialogControl voltControlgrp Prompt: Voltage Controller Parameters
      mask DialogControl Container15currentContGrp Prompt: Current Controller Parameters
      mask Display: image('$imagefile'); % Use "Edit Image" on toolstrip to change.
  Grid-Forming Converter Power Circuit : Subsystem
      mask Display: image('$imagefile'); % Use "Edit Image" on toolstrip to change.
  PU2Hz : Gain  Gain=gridInverter.frequency
  Volt2PU : Gain  Gain=1/base.voltage
  P : PMIOPort  Side=Left
  N : PMIOPort  Port=2  Side=Left
  ABC : PMIOPort  Port=3  Side=Right
  Pmeas : Outport
  Qmeas : Outport  Port=2
  FreqHz : Outport  Port=3
  Vabcmeas : Outport  Port=4
  Iabcmeas : Outport  Port=5
  wires:
  PU2Hz/1 -> FreqHz/1
  Amp2PU/1 -> Iabcmeas/1  "Iabc"
  Grid-Forming Converter Control/1(mabc) -> [mabc]  "mabc"
  [Igabc] -> Grid-Forming Converter Control/3(Igabc)  "Iabc"
  Grid-Forming Converter Control/2(Pmeas) -> Pmeas/1  "Pmeas"
  [mabc] -> Grid-Forming Converter Power Circuit/1(mabc)
  QrefPU/1 -> Grid-Forming Converter Control/2(Qref)
  Grid-Forming Converter Control/3(Qmeas) -> Qmeas/1  "Qmeas"
  Grid-Forming Converter Power Circuit/2(Vabc) -> Volt2PU/1, [Vgabc]
  PrefPU/1 -> Grid-Forming Converter Control/1(Pref)
  [Vgabc] -> Grid-Forming Converter Control/4(Vgabc)  "Vabc"
  Grid-Forming Converter Control/4(fmeas) -> PU2Hz/1  "Freq"
  Volt2PU/1 -> Vabcmeas/1  "Vabc"
  Grid-Forming Converter Power Circuit/1(Iabc) -> [Igabc], Amp2PU/1
  connections:
  ABC/RConn1 -- Grid-Forming Converter Power Circuit/RConn1
  N/RConn1 -- Grid-Forming Converter Power Circuit/LConn2
  P/RConn1 -- Grid-Forming Converter Power Circuit/LConn1

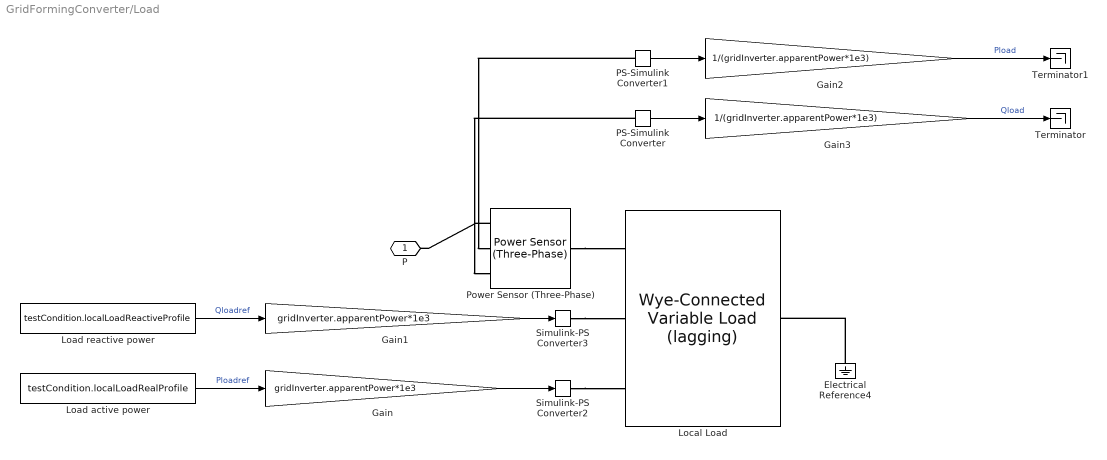
== system GridFormingConverter/Load ==
  Electrical Reference4 : fl_lib/Electrical/Electrical Elements/Electrical Reference
  Gain : Gain  Gain=gridInverter.apparentPower*1e3
  Gain1 : Gain  Gain=gridInverter.apparentPower*1e3
  Gain2 : Gain  Gain=1/(gridInverter.apparentPower*1e3)
  Gain3 : Gain  Gain=1/(gridInverter.apparentPower*1e3)
  Load active power : FromWorkspace  VariableName=testCondition.localLoadRealProfile  SampleTime=localSolverSampleTime  Interpolate=off  OutputAfterFinalValue=Holding final value
  Load reactive power : FromWorkspace  VariableName=testCondition.localLoadReactiveProfile  SampleTime=localSolverSampleTime  Interpolate=off  OutputAfterFinalValue=Holding final value
  Local Load : ee_lib/Passive/RLC Assemblies/Wye-Connected Variable Load (lagging)  VRated=gridInverter.lineRMSVoltage V  FRated=gridInverter.frequency Hz  Pmin=gridInverter.apparentPower*0.05 W  Qmin=gridInverter.apparentPower*0.01 A*V  G_parasitic=1e-6 1/Ohm  I_specify=off  I_priority=None  I=[0, 0, 0] A  I_nominal_specify=off  I_nominal_value=1  I_nominal_unit=A  Phi_specify=off  Phi_priority=None  Phi=[0, 0, 0] Wb  Phi_nominal_specify=off  Phi_nominal_value=1  Phi_nominal_unit=Wb
      settings: InternalSimscapePortConfiguration="{\"Bottom\":[],\"Left\":[{\"id\":\"P\",\"label\":\"P\",\"type\":\"input\"},{\"id\":\"Q\",\"label\":\"Q\",\"type\":\"input\"},{\"id\":\"N\",\"label\":\"~\",\"type\":\"foundation.electrical.three_phase\"}],\"Right\":[{\"id\":\"n\",\"label\":\"n\",\"type\":\"foundation.electrical.electrical\"}],\"Top\":[]}"
  PS-Simulink Converter : nesl_utility/PS-Simulink Converter  PhysicalDomain=network_engine_domain  SubClassName=ps_output  LeftPortType=input  RightPortType=output  PseudoPeriodic=off  Frequencies=[]  VectorFormat=inherit  Unit=inherit  AffineConversion=off
  PS-Simulink Converter1 : nesl_utility/PS-Simulink Converter  PhysicalDomain=network_engine_domain  SubClassName=ps_output  LeftPortType=input  RightPortType=output  PseudoPeriodic=off  Frequencies=[]  VectorFormat=inherit  Unit=inherit  AffineConversion=off
  Power Sensor (Three-Phase) : ee_lib/Sensors & Transducers/Power Sensor (Three-Phase)  load_type=ee.enum.passive.type_balanced.balanced  f0=60 Hz  config=ee.enum.with_neutral.no  rho=1
      settings: InternalSimscapePortConfiguration="{\"Bottom\":[],\"Left\":[{\"id\":\"N1\",\"label\":\"~1\",\"type\":\"foundation.electrical.three_phase\"}],\"Right\":[{\"id\":\"N2\",\"label\":\"~2\",\"type\":\"foundation.electrical.three_phase\"}],\"Top\":[{\"id\":\"Pm\",\"label\":\"P\",\"type\":\"output\"},{\"id\":\"Qm\",\"label\":\"Q\",\"type\":\"output\"}]}"
  Simulink-PS Converter2 : nesl_utility/Simulink-PS Converter  PhysicalDomain=network_engine_domain  SubClassName=ps_input  LeftPortType=input  RightPortType=output  PseudoPeriodic=off  Frequencies=[]  NoiseDistribution=none  NoiseParameters=[]  Unit=1  AffineConversion=off  FilteringAndDerivatives=provide  SimscapeFilterOrder=1  InputFilterTimeConstant=0.001  UdotUserProvided=0
  Simulink-PS Converter3 : nesl_utility/Simulink-PS Converter  PhysicalDomain=network_engine_domain  SubClassName=ps_input  LeftPortType=input  RightPortType=output  PseudoPeriodic=off  Frequencies=[]  NoiseDistribution=none  NoiseParameters=[]  Unit=1  AffineConversion=off  FilteringAndDerivatives=provide  SimscapeFilterOrder=1  InputFilterTimeConstant=0.001  UdotUserProvided=0
  Terminator : Terminator
  Terminator1 : Terminator
  P : PMIOPort  Side=Left
  wires:
  Load reactive power/1 -> Gain1/1  "Qloadref"
  Gain/1 -> Simulink-PS Converter2/1
  Load active power/1 -> Gain/1  "Ploadref"
  Gain1/1 -> Simulink-PS Converter3/1
  PS-Simulink Converter1/1 -> Gain2/1
  PS-Simulink Converter/1 -> Gain3/1
  Gain2/1 -> Terminator1/1  "Pload"
  Gain3/1 -> Terminator/1  "Qload"
  connections:
  Electrical Reference4/LConn1 -- Local Load/RConn1
  Simulink-PS Converter3/RConn1 -- Local Load/LConn2
  Simulink-PS Converter2/RConn1 -- Local Load/LConn1
  Power Sensor (Three-Phase)/LConn1 -- P/RConn1
  Power Sensor (Three-Phase)/RConn1 -- Local Load/LConn3
  PS-Simulink Converter1/LConn1 -- Power Sensor (Three-Phase)/LConn2
  PS-Simulink Converter/LConn1 -- Power Sensor (Three-Phase)/LConn3

== system GridFormingConverter/Power Reference ==
  Active power reference : FromWorkspace  VariableName=testCondition.gfmRealPowerRefProfile  SampleTime=localSolverSampleTime  OutputAfterFinalValue=Holding final value
  Low-Pass Filter (Discrete or Continuous) : eeGeneralControl/Low-Pass Filter (Discrete or Continuous)  K=1  T=5e-2  B=inf  A=-inf  init_option=Inherited from block input  x0=0  Ts=-1
  Low-Pass Filter (Discrete or Continuous)1 : eeGeneralControl/Low-Pass Filter (Discrete or Continuous)  K=1  T=5e-2  B=inf  A=-inf  init_option=Inherited from block input  x0=0  Ts=-1
  Reactive power reference : FromWorkspace  VariableName=testCondition.gfmReactivePowerRefProfile  SampleTime=localSolverSampleTime  OutputAfterFinalValue=Holding final value
  Pref : Outport
  Qref : Outport  Port=2
  wires:
  Active power reference/1 -> Low-Pass Filter (Discrete or Continuous)/1  "Pref"
  Reactive power reference/1 -> Low-Pass Filter (Discrete or Continuous)1/1  "Qref"
  Low-Pass Filter (Discrete or Continuous)/1 -> Pref/1
  Low-Pass Filter (Discrete or Continuous)1/1 -> Qref/1

== system GridFormingConverter/Select the Test Condition ==

== system GridFormingConverter/Transformer 415 V//11 kV ==
  Circuit Breaker : ee_lib/Switches & Breakers/Circuit Breaker (Three-Phase)  R_closed=0.001 Ohm  G_open=1e-6 1/Ohm  threshold=0.5 V  breaker_behavior=ee.enum.switches.breakerBehavior.zeroCrossingEnable
      settings: InternalSimscapePortConfiguration="{\"Bottom\":[],\"Left\":[{\"id\":\"vT\",\"label\":\"vT\",\"type\":\"input\"},{\"id\":\"N1\",\"label\":\"~1\",\"type\":\"foundation.electrical.three_phase\"}],\"Right\":[{\"id\":\"N2\",\"label\":\"~2\",\"type\":\"foundation.electrical.three_phase\"}],\"Top\":[]}"
  Circuit breaker : FromWorkspace  VariableName=testCondition.circuitBreakerTripSignalProfile  SampleTime=localSolverSampleTime  Interpolate=off  OutputAfterFinalValue=Holding final value
  Simulink-PS Converter : nesl_utility/Simulink-PS Converter  PhysicalDomain=network_engine_domain  SubClassName=ps_input  LeftPortType=input  RightPortType=output  PseudoPeriodic=off  Frequencies=[]  NoiseDistribution=none  NoiseParameters=[]  Unit=1  AffineConversion=off  FilteringAndDerivatives=provide  SimscapeFilterOrder=1  InputFilterTimeConstant=0.001  UdotUserProvided=0
  "Transformer " : ee_lib/Passive/Transformers/Two-Winding Transformer (Three-Phase)  SRated=base.power*1e3 A*V  FRated=gridInverter.frequency Hz  Winding1Connection=ee.enum.windingconnection.Yg  VRated1=transformer.primaryRMSVoltage V  Winding2Connection=ee.enum.windingconnection.delta1  VRated2=transformer.secondaryRMSVoltage V  CoreType=ee.enum.coretype.threelimb  pu_Rw1=transformer.PrimaryResistancePU*scrFactorRg  pu_Rw2=transformer.SecondaryResistancePU*scrFactorRg  leakage_reactance_option=ee.enum.transformer_leakage.include  pu_Xl1=transformer.PrimaryReactancePU*scrFactorXg  pu_Xl2=transformer.SecondaryReactancePU*scrFactorXg  magnetizing_resistance_option=ee.enum.transformer_magnetizingResistance.exclude  pu_Rm=500  magnetizing_reactance_option=ee.enum.transformer_magnetizingReactance.exclude  saturation_option=ee.enum.transformer_saturation.exclude  pu_Xm=500  current_data=[0, .002, 1, 2]  magnetic_flux_data=[0, 1.2, 1.5, 1.51]  pu_X0=transformer.PrimaryReactancePU*scrFactorXg*1.05  i1_specify=on  i1_priority=None  i1=[0, 0, 0] A  i1_nominal_specify=off  i1_nominal_value=1  i1_nominal_unit=A  i2_specify=on  i2_priority=None  i2=[0, 0, 0] A  i2_nominal_specify=off  i2_nominal_value=1  i2_nominal_unit=A  phi_specify=off  phi_priority=None  phi=[0, 0, 0]  phi_nominal_specify=off  phi_nominal_value=1  phi_nominal_unit=1  power_dissipated_specify=off  power_dissipated_priority=None  power_dissipated=0 W  power_dissipated_nominal_specify=off  power_dissipated_nominal_value=1  power_dissipated_nominal_unit=W
      settings: InternalSimscapePortConfiguration="{\"Bottom\":[],\"Left\":[{\"id\":\"N1\",\"label\":\"~1\",\"type\":\"foundation.electrical.three_phase\"}],\"Right\":[{\"id\":\"N2\",\"label\":\"~2\",\"type\":\"foundation.electrical.three_phase\"}],\"Top\":[]}"
  ABC1 : PMIOPort  Side=Left
  ABC2 : PMIOPort  Port=2  Side=Right
  wires:
  Circuit breaker/1 -> Simulink-PS Converter/1  "Tripsignal"
  connections:
  "Transformer "/RConn1 -- ABC2/RConn1
  Simulink-PS Converter/RConn1 -- Circuit Breaker/LConn1
  ABC1/RConn1 -- Circuit Breaker/RConn1
  "Transformer "/LConn1 -- Circuit Breaker/LConn2

== system GridFormingConverter/Transmission Line ==
  Transmission Line : ee_lib/Passive/RLC Assemblies/RLC (Three-Phase)  port_option=ee.enum.threePhasePort.composite  component_structure=ee.enum.rlc.structure.SeriesRL  R=TransmissionLine.R*scrFactorRg Ohm  L=TransmissionLine.L*scrFactorXg H  C=1e-6 F  R_parasitic=0 Ohm  G_parasitic=1e-5 1/Ohm  IL_specify=off  IL_priority=High  IL=[0, 0, 0] A  IL_nominal_specify=off  IL_nominal_value=1  IL_nominal_unit=A  VC_specify=off  VC_priority=High  VC=[0, 0, 0] V  VC_nominal_specify=off  VC_nominal_value=1  VC_nominal_unit=V
      settings: InternalSimscapePortConfiguration="{\"Bottom\":[],\"Left\":[{\"id\":\"N1\",\"label\":\"~1\",\"type\":\"foundation.electrical.three_phase\"}],\"Right\":[{\"id\":\"N2\",\"label\":\"~2\",\"type\":\"foundation.electrical.three_phase\"}],\"Top\":[]}"
  ABC1 : PMIOPort  Side=Left
  ABC2 : PMIOPort  Port=2  Side=Right
  connections:
  Transmission Line/RConn1 -- ABC2/RConn1
  ABC1/RConn1 -- Transmission Line/LConn1

== system GridFormingConverter/Grid-Forming Converter/Grid-Forming Converter Control ==
  Pref : Inport
  Qref : Inport  Port=2
  Igabc : Inport  Port=3
  Vgabc : Inport  Port=4
  Current Limiting : Subsystem
  Grid Voltage Reactive Power Support : Subsystem
  Measurement : Subsystem
      mask Display: image('$imagefile'); % Use "Edit Image" on toolstrip to change.
  Power Control : Subsystem
  Rate Transition3 : RateTransition
  VoltageCurrentControl : Subsystem
      settings: PortSchema="{\"entries\":[{\"content\":{\"sides\":[{\"content\":{\"connectorIds\":[\"In1\",\"In2\"]},\"type\":\"ConnectorPlacement.EquallySpacedRectSide\",\"uuid\":\"0bf15a12-7bc0-47e4-89bd-435769673763\"},{\"content\":{\"connectorIds\":[\"Out1\"],\"side\":\"RIGHT\"},\"type\":\"ConnectorPlacement.EquallySpacedRectSide\",\"uuid\":\"44a15d74-8878-4ec6-abe4-be0b1b609519\"},{\"content\":{\"connectorIds\":[\"In3\"],\"side\":\"TOP\"},\"type\":\"ConnectorPlacement.EquallySpacedRectSide\",\"uuid\":\"7a96781e-5638-4b2a-8101-d5785aae9f0f\"}]},\"type\":\"ConnectorPlacement.EquallySpacedConnector\",\"uuid\":\"4b3373ad-cf20-4175-894e-3bd1604dd0ce\"}],\"packageUris\":[\"http://schema.mathworks.com/mf0/Connector/R2020b\"],\"version\":\"1.0\"}"
  mabc : Outport
  Pmeas : Outport  Port=2
  Qmeas : Outport  Port=3
  fmeas : Outport  Port=4
  wires:
  VoltageCurrentControl/1(mabc) -> mabc/1
  Vgabc/1 -> Measurement/1(Vgabcc)
  Igabc/1 -> Measurement/2(Igabc)
  Measurement/2(Pmeas) -> Pmeas/1
  Measurement/3(Qmeas) -> Qmeas/1
  Measurement/1(measure) -> Rate Transition3/1
  Power Control/3(angle) -> Measurement/3(Angle)
  Power Control/1(reactiveControl) -> Current Limiting/2(reactiveControl)
  Current Limiting/1(currentLimiting) -> VoltageCurrentControl/1(currentLimiting)
  Qref/1 -> Grid Voltage Reactive Power Support/3(QrefInput)
  Pref/1 -> Grid Voltage Reactive Power Support/2(PrefInput)
  Grid Voltage Reactive Power Support/1(Pref) -> Power Control/2(Pref)
  Grid Voltage Reactive Power Support/2(Qref) -> Power Control/3(Qref)
  Measurement/4(fmeas) -> fmeas/1
  Rate Transition3/1 -> Current Limiting/1(measure), VoltageCurrentControl/3(measure), Power Control/1(measure), Grid Voltage Reactive Power Support/1(measure)
  Power Control/2(activeControl) -> VoltageCurrentControl/2(activeControl)
